simulink model "TrayectoriaPurePursuitSM"  (R2023b)
settings: Solver=VariableStepAuto  StartTime=0.0  StopTime=150  RelTol=1e-3
undefined symbols (not defined in the file): d, DiscIntNeverNeededParam
libraries: slpidlib x1
settings Model: Creator=keanu  LastModifiedBy=keanu

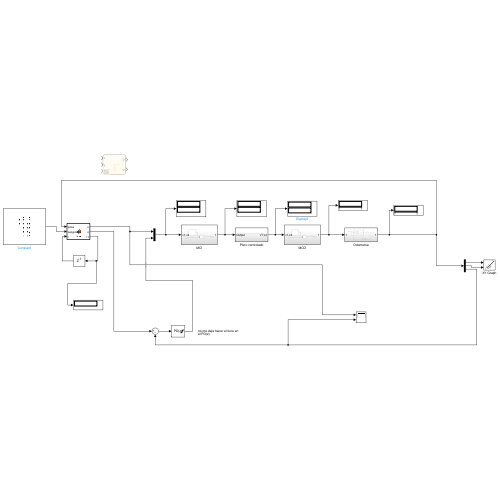
[thumbnail: Simulink's stored preview of the top-level diagram]
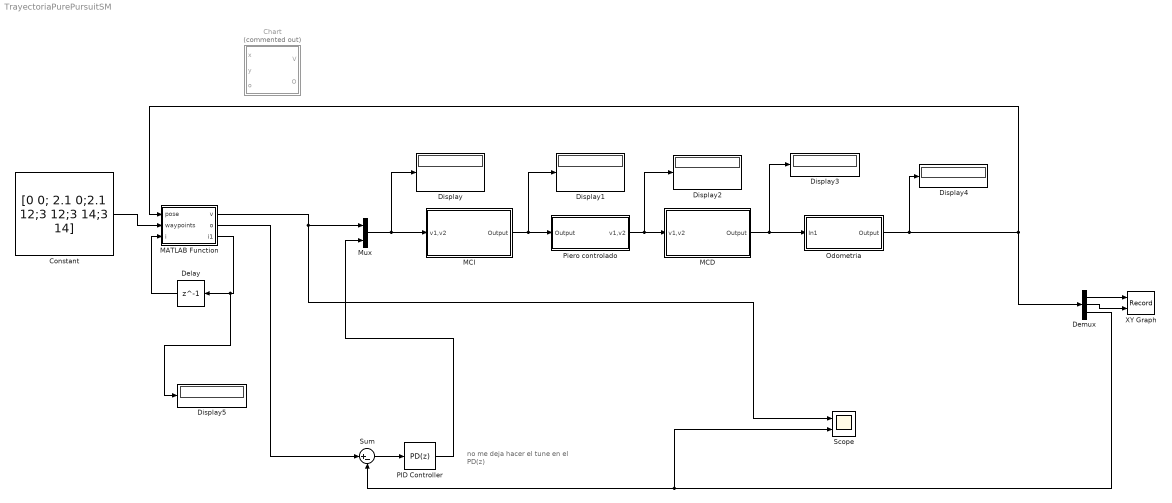
== system TrayectoriaPurePursuitSM ==
  note: no me deja hacer el tune en el PD(z)
  Chart : Stateflow chart  Commented=on  TreatAsAtomicUnit=on
  Constant : Constant  Value=[0 0; 2.1 0;2.1 12;3 12;3 14;3 14]
  Delay : Delay  DelayLength=1
  Demux : Demux  Outputs=3
  Display{,1..5} (6 alike) : Display
  MATLAB Function : MATLAB Function  TreatAsAtomicUnit=on
  MCD : Subsystem
  MCI : Subsystem
  Mux : Mux  Inputs=2
  Odometria : Subsystem
  PID Controller : slpidlib/PID Controller  Controller=PD  Form=Parallel  TimeDomain=Discrete-time  UseExternalTs=off  SampleTime=-1  IntegratorMethod=Forward Euler  FilterMethod=Forward Euler  ControllerParametersSource=internal  P=3.29979459563487  I=0  UseKiTs=off  D=0.42470318788058  N=5.41551557604445  UseFilter=on  TunerSelectOption=Transfer Function Based (PID Tuner App)  InitialConditionSource=internal  InitialConditionForIntegrator=0  InitialConditionForFilter=0  DifferentiatorICPrevScaledInput=0  ExternalReset=none  TrackingMode=off  Kt=1  LimitOutput=on  SatLimitsSource=internal  UpperSaturationLimit=inf  LowerSaturationLimit=-inf  LinearizeAsGain=on  AntiWindupMode=none  Kb=1  LimitIntegrator=off  UpperIntegratorSaturationLimit=inf  LowerIntegratorSaturationLimit=-inf  POutMin=[]  POutMax=[]  IOutMin=[]  IOutMax=[]  DOutMin=[]  DOutMax=[]  NOutMin=[]  NOutMax=[]  SumOutMin=[]  SumOutMax=[]  SaturationOutMin=[]  SaturationOutMax=[]  PParamMin=[]  PParamMax=[]  IParamMin=[]  IParamMax=[]  DParamMin=[]  DParamMax=[]  NParamMin=[]  NParamMax=[]  KbParamMin=[]  KbParamMax=[]  KtParamMin=[]  KtParamMax=[]  KbOutMin=[]  KbOutMax=[]  KtOutMin=[]  KtOutMax=[]  IntegratorOutMin=[]  IntegratorOutMax=[]  FilterOutMin=[]  FilterOutMax=[]  SumI1OutMin=[]  SumI1OutMax=[]  SumI2OutMin=[]  SumI2OutMax=[]  SumI3OutMin=[]  SumI3OutMax=[]  SumI4OutMin=[]  SumI4OutMax=[]  SumDOutMin=[]  SumDOutMax=[]  DifferentiatorOutMin=[]  DifferentiatorOutMax=[]  FilterDiffOutCoefMin=[]  FilterDiffOutCoefMax=[]  ReciprocalOutMin=[]  ReciprocalOutMax=[]  SumDenOutMin=[]  SumDenOutMax=[]  SumNumOutMin=[]  SumNumOutMax=[]  DivideOutMin=[]  DivideOutMax=[]  UdiffTsProdOutMin=[]  UdiffTsProdOutMax=[]  NTsProdOutMin=[]  NTsProdOutMax=[]  UintegralTsProdOutMin=[]  UintegralTsProdOutMax=[]  UngainTsProdOutMin=[]  UngainTsProdOutMax=[]  ClampingZeroOutDataTypeStr=Inherit: Inherit via back propagation  ClampingZeroOutMin=[]  ClampingZeroOutMax=[]  FilterDenConstantOutDataTypeStr=Inherit: Inherit via back propagation  FilterDenConstantOutMin=[]  FilterDenConstantOutMax=[]  PCopyOutDataTypeStr=Inherit: Inherit via back propagation  PCopyOutMin=[]  PCopyOutMax=[]  NCopyOutDataTypeStr=Inherit: Inherit via back propagation  NCopyOutMin=[]  NCopyOutMax=[]  IntegratorContinuousStateAttributes=''  IntegratorStateMustResolveToSignalObject=off  IntegratorRTWStateStorageClass=Auto  FilterContinuousStateAttributes=''  FilterStateMustResolveToSignalObject=off  FilterRTWStateStorageClass=Auto  ParallelPVariant=InternalParameters  IdealPVariant=Disabled  IVariant=Disabled  DVariant=InternalParameters  IntegratorVariant=Disabled  SatVariant=Enabled  AWVariant=Disabled  PCopyVariant=Disabled  TRVariant=Disabled  FdbkBlocksVariant=Forward  IdealPFdbkVariant=Disabled  SatFdbkVariant=Disabled  DerivativeFilterVariant=ForwardEulerFilter  NVariant=InternalParameters  NCopyVariant=Disabled  FilterICVariant=InternalICsFilter  IntegratorICVariant=Disabled  ExternalResetVariant=Disabled  TRSumVariant=Passthrough  SumFdbkVariant=Disabled  SumVariant=Sum_PD  TsampFilterVariant=InternalTs  TsampNgainVariant=Passthrough  TsampIntegralVariant=Disabled_SignalSpec  ExternalSaturationOutDataTypeStr=Inherit: Same as second input
  Piero controlado : Subsystem
  Scope : Scope  NumInputPorts=2
  Sum : Sum  Inputs=|+-
  XY Graph : Record  FileSettingsInternal="{\"entries\":[{\"content\":{\"excelSettings\":{\"content\":{},\"type\":\"Streamout.ExcelSettings\"}},\"type\":\"Streamout.FileSettingStorage\",\"uuid\":\"\"}],\"packageUris\":[\"http:\\/\\/schema.mathworks.com\\/mf0\\/streamout_blocks\\/R2020a\"],\"version\":\"1.0\"}"  Layout=[1 1]  SignalsInternal="{\"entries\":[{\"content\":{\"signals\":[{\"content\":{\"blockPath\":[],\"dimensions\":[1],\"domain\":\"\",\"lineColor\":\"#edb120\",\"port\":1,\"sid\":[\"\"],\"signalID\":1,\"signalName\":\"Demux:1\"},\"type\":\"RecordBlkView.Signal\",\"uuid\":\"\"},{\"content\":{\"blockPath\":[],\"dimensions\":[1],\"domain\":\"\",\"lineColor\":\"#7e2f8e\",\"port\":2,\"sid\":[\"\"],\"signalID\":2,\"signalName\":\"Demux:2\"},\"type\":\"RecordBlkView.Signal\",\"uuid\":\"\"}]},\"type\":\"RecordBlkView.InputSignals\",\"uuid\":\"\"}],\"packageUris\":[\"http:\\/\\/schema.mathworks.com\\/mf0\\/streamout_blocks\\/R2020a\"],\"version\":\"1.0\"}"  VisualizationBindings="{\"xyplotplugin\":{\"info\":[{\"series\":[],\"subplotID\":1}]}}"  CompatibilityTag=XY
  wires:
  MCD/1(Output) -> Display3/1, Odometria/1(In1)
  Mux/1 -> Display/1, MCI/1(v1,v2)
  MCI/1(Output) -> Piero controlado/1(Output), Display1/1
  Odometria/1(Output) -> Display4/1, MATLAB Function/1(pose), Demux/1
  Demux/1 -> XY Graph/1
  Demux/2 -> XY Graph/2
  Sum/1 -> PID Controller/1
  Demux/3 -> Scope/2, Sum/2
  MATLAB Function/1(v) -> Scope/1, Mux/1
  MATLAB Function/3(i1) -> Display5/1, Delay/1
  Delay/1 -> MATLAB Function/3(i)
  Piero controlado/1(v1,v2) -> Display2/1, MCD/1(v1,v2)
  MATLAB Function/2(o) -> Sum/1
  PID Controller/1 -> Mux/2
  Constant/1 -> MATLAB Function/2(waypoints)

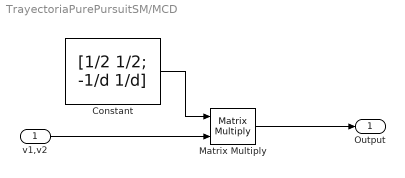
== system TrayectoriaPurePursuitSM/MCD ==
  v1,v2 : Inport
  Constant : Constant  Value=[1/2 1/2; -1/d 1/d]
  Matrix Multiply : Product  Multiplication=Matrix(*)
  Output : Outport
  wires:
  Matrix Multiply/1 -> Output/1
  v1,v2/1 -> Matrix Multiply/2
  Constant/1 -> Matrix Multiply/1

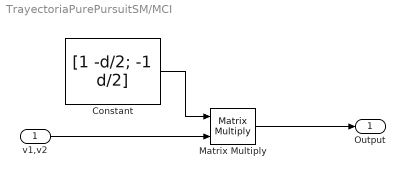
== system TrayectoriaPurePursuitSM/MCI ==
  v1,v2 : Inport
  Constant : Constant  Value=[1 -d/2; -1 d/2]
  Matrix Multiply : Product  Multiplication=Matrix(*)
  Output : Outport
  wires:
  Constant/1 -> Matrix Multiply/1
  v1,v2/1 -> Matrix Multiply/2
  Matrix Multiply/1 -> Output/1

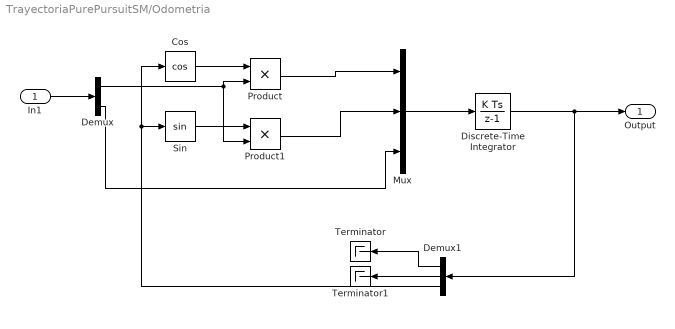
== system TrayectoriaPurePursuitSM/Odometria ==
  In1 : Inport
  Cos : Trigonometry  Operator=cos
  Demux : Demux  Outputs=2
  Demux1 : Demux  Outputs=3
  Discrete-Time Integrator : DiscreteIntegrator  SampleTime=-1  ICPrevOutput=DiscIntNeverNeededParam  ICPrevScaledInput=DiscIntNeverNeededParam
  Mux : Mux  Inputs=3
  Product : Product
  Product1 : Product
  Sin : Trigonometry
  Terminator : Terminator
  Terminator1 : Terminator
  Output : Outport
  wires:
  Discrete-Time Integrator/1 -> Demux1/1, Output/1
  Product1/1 -> Mux/2
  In1/1 -> Demux/1
  Cos/1 -> Product/1
  Demux/2 -> Mux/3
  Demux1/3 -> Sin/1, Cos/1
  Product/1 -> Mux/1
  Demux1/2 -> Terminator1/1
  Sin/1 -> Product1/1
  Mux/1 -> Discrete-Time Integrator/1
  Demux/1 -> Product1/2, Product/2
  Demux1/1 -> Terminator/1

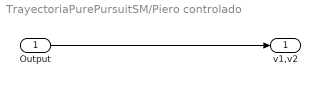
== system TrayectoriaPurePursuitSM/Piero controlado ==
  Output : Inport
  v1,v2 : Outport
  wires:
  Output/1 -> v1,v2/1

== matlab function TrayectoriaPurePursuitSM/MATLAB Function ==
  data: v output double size=1; pose input; o output size=1; waypoints input; i1 output size=1; i input size=1
function [v, o, i1] = fcn(pose, waypoints, i)

LA=0.30;
%if isempty (indice)
  %  persistent indice=0;
%end
v = 0.205;
i=i+1;
i1=0;
x=pose(1);
y=pose(2);
O=pose(3);

if(length(waypoints) >= i)

    distancia=sqrt((waypoints(i,1)-x)^2 +(waypoints(i,2)-y)^2);

    while (distancia < LA) && (length(waypoints)>i)
        i=i+1;
        distancia=sqrt((waypoints(i,1)-x)^2 +(waypoints(i,2)-y)^2);
        v=0.1;
    end
    o=atan2(waypoints(i,2)-y,waypoints(i,1)-x);
else
    o=pose(3);
    v=0;
end
if(length(waypoints) > i)
    i1=i-1;
else
    i1=i;
end

== stateflow chart TrayectoriaPurePursuitSM/Chart ==
  state Paro
    V=0;
    O=pi/2;
  state Recto2
    V=0.205;
    O=pi/2;
  state GiroDcha
    V=0.10;
    O=0;
  state Recto1
    V=0.205;
    O=0;
  state GiroIzq1
    V=0.10;
    O=pi/2;
  state Recto
    V=0.205;
    O=pi/2;
  state Inicio
    V=0;
    O=0;
    w=0;
  state Marcha
    V=0.205;
    O=0;
  state GiroIzq
    V=0.10;
    O=pi/2;
  Recto2 -> Paro : [y>14]
  GiroIzq1 -> Recto2 : [o>pi/2]
  Recto1 -> GiroIzq1 : [x>3]
  GiroDcha -> Recto1 : [o>0]
  Recto -> GiroDcha : [y>12]
  GiroIzq -> Recto : [o>pi/2]
  (default) -> Inicio
  Inicio -> Marcha : [after(1,sec)]
  Marcha -> GiroIzq : [x>1.7]
  data: V output double size=1; x input double size=1; y input double size=1; o input double size=1; O output
